simulink model "draft3"  (R2023a)
settings: Solver=VariableStepAuto  StartTime=0.0  StopTime=inf  FixedStep=0.0001  MaxStep=0.2  RelTol=1e-3  AbsTol=1e-3  EnableMultiTasking=on
model workspace (MAT data in the model file):
  c = 0.1
  k : Simulink.Parameter (value not decoded)
libraries: sm_lib x40, nesl_utility x35, simulink_extras x2, fl_lib x1
(part 3 of 3)

== system draft3/Thoracic Spine with rigid joints/T7 ==
  T7 : sm_lib/Body Elements/File Solid  ExtGeomFileName=C:\Users\siril\OneDrive\Desktop\TIM-Control\Matlab\Simscape models\CAD - with COM\T7_.step  UnitType=FromFile  ExtGeomFileUnits=m  StepReaderType=HEX  ExportConvexHullGeometry=off  InertiaType=CalculateFromGeometry  Mass=1  MassUnits=kg  CenterOfMass=[0 0 0]  CenterOfMassUnits=m  MomentsOfInertia=[1 1 1]  MomentsOfInertiaUnits=kg*m^2  ProductsOfInertia=[0 0 0]  ProductsOfInertiaUnits=kg*m^2  BasedOnType=Density  Density=0.99  DensityUnits=g/cm^3  DoExposeReferenceFrame=on  SerializedFrames=<Frames><Frame><Id>Frame1</Id><Value><Name>COM</Name><Origin><Source>CenterOfMassFrame</Source><FeatureName></FeatureName></Origin><PrimaryAxis><DefinedDirection>+Z</DefinedDirection><Source>ReferenceFrame</Source><SourceDirection>+Z</SourceDirection><FeatureName></FeatureName></PrimaryAxis><SecondaryAxis><DefinedDirection>+X</DefinedDirection><Source>ReferenceFrame</Source><SourceDirection>+X</SourceDirection><FeatureName></FeatureName></SecondaryAxis></Value></Frame><Frame><Id>Frame2</Id><Value><Name>to T8</Name><Origin><Source>GeometricFeature</Source><FeatureName>planar surface 5</FeatureName></Origin><PrimaryAxis><DefinedDirection>+X</DefinedDirection><Source>GeometricFeature</Source><SourceDirection>+Z</SourceDirection><FeatureName>planar surface 5</FeatureName></PrimaryAxis><SecondaryAxis><DefinedDirection>+Y</DefinedDirection><Source>ReferenceFrame</Source><SourceDirection>-X</SourceDirection><FeatureName></FeatureName></SecondaryAxis></Value></Frame><Frame><Id>Frame3</Id><Value><Name>to T6</Name><Origin><Source>GeometricFeature</Source><FeatureName>planar surface 10</FeatureName></Origin><PrimaryAxis><DefinedDirection>+Z</DefinedDirection><Source>ReferenceFrame</Source><SourceDirection>+Z</SourceDirection><FeatureName></FeatureName></PrimaryAxis><SecondaryAxis><DefinedDirection>+X</DefinedDirection><Source>ReferenceFrame</Source><SourceDirection>+X</SourceDirection><FeatureName></FeatureName></SecondaryAxis></Value></Frame></Frames>  GraphicType=FromGeometry  MarkerShape=Sphere  MarkerSize=10  GraphicVisPropType=SimpleVisualProperties  GraphicDiffuseColor=[0.5 0.5 0.5]  GraphicSpecularColor=[0.5 0.5 0.5 1.0]  GraphicAmbientColor=[0.15 0.15 0.15 1.0]  GraphicEmissiveColor=[0.0 0.0 0.0 1.0]  GraphicShininess=75  GraphicOpacity=1.0
  Weld Joint : sm_lib/Joints/Weld Joint  JointMode=Normal  SenseConstraintForce=off  SenseConstraintForceX=off  SenseConstraintForceY=off  SenseConstraintForceZ=off  SenseConstraintTorque=off  SenseConstraintTorqueX=off  SenseConstraintTorqueY=off  SenseConstraintTorqueZ=off  SenseTotalForce=off  SenseTotalForceX=off  SenseTotalForceY=off  SenseTotalForceZ=off  SenseTotalTorque=off  SenseTotalTorqueX=off  SenseTotalTorqueY=off  SenseTotalTorqueZ=off  CompositeWrenchDir=FollowerOnBase  CompositeWrenchFrame=BaseFrame
  to T8 : PMIOPort  Side=Left
  T7 COM : PMIOPort  Port=2  Side=Left
  T7 R : PMIOPort  Port=3  Side=Right
  to T6 : PMIOPort  Port=4  Side=Right
  connections:
  T7 COM/RConn1 -- T7/LConn1
  T7/RConn1 -- T7 R/RConn1
  to T6/RConn1 -- T7/RConn2
  to T8/RConn1 -- Weld Joint/LConn1
  Weld Joint/RConn1 -- T7/LConn2

== system draft3/Thoracic Spine with rigid joints/T8 ==
  T8 : sm_lib/Body Elements/File Solid  ExtGeomFileName=C:\Users\siril\OneDrive\Desktop\TIM-Control\Matlab\Simscape models\CAD - with COM\T8_.step  UnitType=FromFile  ExtGeomFileUnits=m  StepReaderType=HEX  ExportConvexHullGeometry=off  InertiaType=CalculateFromGeometry  Mass=1  MassUnits=kg  CenterOfMass=[0 0 0]  CenterOfMassUnits=m  MomentsOfInertia=[1 1 1]  MomentsOfInertiaUnits=kg*m^2  ProductsOfInertia=[0 0 0]  ProductsOfInertiaUnits=kg*m^2  BasedOnType=Density  Density=0.99  DensityUnits=g/cm^3  DoExposeReferenceFrame=on  SerializedFrames=<Frames><Frame><Id>Frame1</Id><Value><Name>COM</Name><Origin><Source>CenterOfMassFrame</Source><FeatureName></FeatureName></Origin><PrimaryAxis><DefinedDirection>+Z</DefinedDirection><Source>ReferenceFrame</Source><SourceDirection>+Z</SourceDirection><FeatureName></FeatureName></PrimaryAxis><SecondaryAxis><DefinedDirection>+X</DefinedDirection><Source>ReferenceFrame</Source><SourceDirection>+X</SourceDirection><FeatureName></FeatureName></SecondaryAxis></Value></Frame><Frame><Id>Frame2</Id><Value><Name>to T9</Name><Origin><Source>GeometricFeature</Source><FeatureName>planar surface 5</FeatureName></Origin><PrimaryAxis><DefinedDirection>+X</DefinedDirection><Source>GeometricFeature</Source><SourceDirection>+Z</SourceDirection><FeatureName>planar surface 5</FeatureName></PrimaryAxis><SecondaryAxis><DefinedDirection>+Y</DefinedDirection><Source>ReferenceFrame</Source><SourceDirection>-X</SourceDirection><FeatureName></FeatureName></SecondaryAxis></Value></Frame><Frame><Id>Frame3</Id><Value><Name>to T7</Name><Origin><Source>GeometricFeature</Source><FeatureName>planar surface 20</FeatureName></Origin><PrimaryAxis><DefinedDirection>+X</DefinedDirection><Source>GeometricFeature</Source><SourceDirection>+Z</SourceDirection><FeatureName>planar surface 20</FeatureName></PrimaryAxis><SecondaryAxis><DefinedDirection>+Y</DefinedDirection><Source>ReferenceFrame</Source><SourceDirection>-X</SourceDirection><FeatureName></FeatureName></SecondaryAxis></Value></Frame></Frames>  GraphicType=FromGeometry  MarkerShape=Sphere  MarkerSize=10  GraphicVisPropType=SimpleVisualProperties  GraphicDiffuseColor=[0.5 0.5 0.5]  GraphicSpecularColor=[0.5 0.5 0.5 1.0]  GraphicAmbientColor=[0.15 0.15 0.15 1.0]  GraphicEmissiveColor=[0.0 0.0 0.0 1.0]  GraphicShininess=75  GraphicOpacity=1.0
  Weld Joint : sm_lib/Joints/Weld Joint  JointMode=Normal  SenseConstraintForce=off  SenseConstraintForceX=off  SenseConstraintForceY=off  SenseConstraintForceZ=off  SenseConstraintTorque=off  SenseConstraintTorqueX=off  SenseConstraintTorqueY=off  SenseConstraintTorqueZ=off  SenseTotalForce=off  SenseTotalForceX=off  SenseTotalForceY=off  SenseTotalForceZ=off  SenseTotalTorque=off  SenseTotalTorqueX=off  SenseTotalTorqueY=off  SenseTotalTorqueZ=off  CompositeWrenchDir=FollowerOnBase  CompositeWrenchFrame=BaseFrame
  to T9 : PMIOPort  Side=Left
  T8 COM : PMIOPort  Port=2  Side=Left
  T8 R : PMIOPort  Port=3  Side=Right
  to T7 : PMIOPort  Port=4  Side=Right
  connections:
  to T7/RConn1 -- T8/RConn2
  T8/RConn1 -- T8 R/RConn1
  T8 COM/RConn1 -- T8/LConn1
  to T9/RConn1 -- Weld Joint/LConn1
  Weld Joint/RConn1 -- T8/LConn2

== system draft3/Thoracic Spine with rigid joints/T9 ==
  T9 : sm_lib/Body Elements/File Solid  ExtGeomFileName=C:\Users\siril\OneDrive\Desktop\TIM-Control\Matlab\Simscape models\CAD - with COM\T9_.step  UnitType=FromFile  ExtGeomFileUnits=m  StepReaderType=HEX  ExportConvexHullGeometry=off  InertiaType=CalculateFromGeometry  Mass=1  MassUnits=kg  CenterOfMass=[0 0 0]  CenterOfMassUnits=m  MomentsOfInertia=[1 1 1]  MomentsOfInertiaUnits=kg*m^2  ProductsOfInertia=[0 0 0]  ProductsOfInertiaUnits=kg*m^2  BasedOnType=Density  Density=0.99  DensityUnits=g/cm^3  DoExposeReferenceFrame=on  SerializedFrames=<Frames><Frame><Id>Frame1</Id><Value><Name>COM</Name><Origin><Source>CenterOfMassFrame</Source><FeatureName></FeatureName></Origin><PrimaryAxis><DefinedDirection>+Z</DefinedDirection><Source>ReferenceFrame</Source><SourceDirection>+Z</SourceDirection><FeatureName></FeatureName></PrimaryAxis><SecondaryAxis><DefinedDirection>+X</DefinedDirection><Source>ReferenceFrame</Source><SourceDirection>+X</SourceDirection><FeatureName></FeatureName></SecondaryAxis></Value></Frame><Frame><Id>Frame2</Id><Value><Name>to T10</Name><Origin><Source>GeometricFeature</Source><FeatureName>planar surface 5</FeatureName></Origin><PrimaryAxis><DefinedDirection>+X</DefinedDirection><Source>GeometricFeature</Source><SourceDirection>+Z</SourceDirection><FeatureName>planar surface 5</FeatureName></PrimaryAxis><SecondaryAxis><DefinedDirection>+Y</DefinedDirection><Source>ReferenceFrame</Source><SourceDirection>-X</SourceDirection><FeatureName></FeatureName></SecondaryAxis></Value></Frame><Frame><Id>Frame3</Id><Value><Name>to T8</Name><Origin><Source>GeometricFeature</Source><FeatureName>planar surface 15</FeatureName></Origin><PrimaryAxis><DefinedDirection>+X</DefinedDirection><Source>GeometricFeature</Source><SourceDirection>+Z</SourceDirection><FeatureName>planar surface 15</FeatureName></PrimaryAxis><SecondaryAxis><DefinedDirection>+Y</DefinedDirection><Source>ReferenceFrame</Source><SourceDirection>-X</SourceDirection><FeatureName></FeatureName></SecondaryAxis></Value></Frame></Frames>  GraphicType=FromGeometry  MarkerShape=Sphere  MarkerSize=10  GraphicVisPropType=SimpleVisualProperties  GraphicDiffuseColor=[0.5 0.5 0.5]  GraphicSpecularColor=[0.5 0.5 0.5 1.0]  GraphicAmbientColor=[0.15 0.15 0.15 1.0]  GraphicEmissiveColor=[0.0 0.0 0.0 1.0]  GraphicShininess=75  GraphicOpacity=1.0
  Weld Joint : sm_lib/Joints/Weld Joint  JointMode=Normal  SenseConstraintForce=off  SenseConstraintForceX=off  SenseConstraintForceY=off  SenseConstraintForceZ=off  SenseConstraintTorque=off  SenseConstraintTorqueX=off  SenseConstraintTorqueY=off  SenseConstraintTorqueZ=off  SenseTotalForce=off  SenseTotalForceX=off  SenseTotalForceY=off  SenseTotalForceZ=off  SenseTotalTorque=off  SenseTotalTorqueX=off  SenseTotalTorqueY=off  SenseTotalTorqueZ=off  CompositeWrenchDir=FollowerOnBase  CompositeWrenchFrame=BaseFrame
  to T10 : PMIOPort  Side=Left
  T9 COM : PMIOPort  Port=2  Side=Left
  T9 R : PMIOPort  Port=3  Side=Right
  to T8 : PMIOPort  Port=4  Side=Right
  connections:
  T9 COM/RConn1 -- T9/LConn1
  T9/RConn1 -- T9 R/RConn1
  to T8/RConn1 -- T9/RConn2
  to T10/RConn1 -- Weld Joint/LConn1
  Weld Joint/RConn1 -- T9/LConn2

== matlab function draft3/L1/LB torque feedback L4/peacewise torque profile4 ==
  data: u input; torque output
function torque = T(u)
torque = 0;
if (u >= 15)
    torque= -0.0015*1*(57.295*15)^4 + 0.1326*(57.295*15)^3 -0.3477*(57.295*15)^2 + 0.499*(57.295*15);
 
elseif (u >= -15 && u<= 15)
    torque= -0.0015*(57.295*u)^4 + 0.1326*(57.295*u)^3 -0.3477*(57.295*u)^2 + 0.499*(57.295*u)   ;
    
elseif (u <= -15)
   torque= -0.0015*1*(57.295*-15)^4 + 0.1326*(57.295*-15)^3 -0.3477*(57.295*-15)^2 + 0.499*(57.295*-15);
end

== matlab function draft3/L5/FE torque feedback L5/peacewise torque profile (+- 15 deg) ==
  data: u input; torque output
function torque = T(u)
torque = 0;
if (u >= 15)
    torque= -0.0015*1*(57.295*15)^4 + 0.1326*(57.295*15)^3 -0.3477*(57.295*15)^2 + 0.499*(57.295*15);
 
elseif (u >= -15 && u<= 15)
    torque= -0.0015*(57.295*u)^4 + 0.1326*(57.295*u)^3 -0.3477*(57.295*u)^2 + 0.499*(57.295*u)   ;
    
elseif (u <= -15)
   torque= -0.0015*1*(57.295*-15)^4 + 0.1326*(57.295*-15)^3 -0.3477*(57.295*-15)^2 + 0.499*(57.295*-15);
end

== matlab function draft3/L5/LB torque feedback L5/peacewise torque profile2 ==
  data: u input; torque output
function torque = T(u)
torque = 0;
if (u >= 15)
    torque= -0.0015*1*(57.295*15)^4 + 0.1326*(57.295*15)^3 -0.3477*(57.295*15)^2 + 0.499*(57.295*15);
 
elseif (u >= -15 && u<= 15)
    torque= -0.0015*(57.295*u)^4 + 0.1326*(57.295*u)^3 -0.3477*(57.295*u)^2 + 0.499*(57.295*u)   ;
    
elseif (u <= -15)
   torque= -0.0015*1*(57.295*-15)^4 + 0.1326*(57.295*-15)^3 -0.3477*(57.295*-15)^2 + 0.499*(57.295*-15);
end

== matlab function draft3/L5/AR torque feedback L5/peacewise torque profile3 ==
  data: u input; torque output
function torque = T(u)
torque = 0;
if (u >= 15)
    torque= -0.0015*1*(57.295*15)^4 + 0.1326*(57.295*15)^3 -0.3477*(57.295*15)^2 + 0.499*(57.295*15);
 
elseif (u >= -15 && u<= 15)
    torque= -0.0015*(57.295*u)^4 + 0.1326*(57.295*u)^3 -0.3477*(57.295*u)^2 + 0.499*(57.295*u)   ;
    
elseif (u <= -15)
   torque= -0.0015*1*(57.295*-15)^4 + 0.1326*(57.295*-15)^3 -0.3477*(57.295*-15)^2 + 0.499*(57.295*-15);
end

== matlab function draft3/L4/LB torque feedback L4/peacewise torque profile4 ==
  data: u input; torque output
function torque = T(u)
torque = 0;
if (u >= 15)
    torque= -0.0015*1*(57.295*15)^4 + 0.1326*(57.295*15)^3 -0.3477*(57.295*15)^2 + 0.499*(57.295*15);
 
elseif (u >= -15 && u<= 15)
    torque= -0.0015*(57.295*u)^4 + 0.1326*(57.295*u)^3 -0.3477*(57.295*u)^2 + 0.499*(57.295*u)   ;
    
elseif (u <= -15)
   torque= -0.0015*1*(57.295*-15)^4 + 0.1326*(57.295*-15)^3 -0.3477*(57.295*-15)^2 + 0.499*(57.295*-15);
end

== matlab function draft3/L4/AR torque feedback L4/peacewise torque profile5 ==
  data: u input; torque output
function torque = T(u)
torque = 0;
if (u >= 15)
    torque= -0.0015*1*(57.295*15)^4 + 0.1326*(57.295*15)^3 -0.3477*(57.295*15)^2 + 0.499*(57.295*15);
 
elseif (u >= -15 && u<= 15)
    torque= -0.0015*(57.295*u)^4 + 0.1326*(57.295*u)^3 -0.3477*(57.295*u)^2 + 0.499*(57.295*u)   ;
    
elseif (u <= -15)
   torque= -0.0015*1*(57.295*-15)^4 + 0.1326*(57.295*-15)^3 -0.3477*(57.295*-15)^2 + 0.499*(57.295*-15);
end

== matlab function draft3/L3/AR torque feedback L4/peacewise torque profile5 ==
  data: u input; torque output
function torque = T(u)
torque = 0;
if (u >= 15)
    torque= -0.0015*1*(57.295*15)^4 + 0.1326*(57.295*15)^3 -0.3477*(57.295*15)^2 + 0.499*(57.295*15);
 
elseif (u >= -15 && u<= 15)
    torque= -0.0015*(57.295*u)^4 + 0.1326*(57.295*u)^3 -0.3477*(57.295*u)^2 + 0.499*(57.295*u)   ;
    
elseif (u <= -15)
   torque= -0.0015*1*(57.295*-15)^4 + 0.1326*(57.295*-15)^3 -0.3477*(57.295*-15)^2 + 0.499*(57.295*-15);
end

== matlab function draft3/L3/FE torque feedback L4/peacewise torque profile1 ==
  data: u input; torque output
function torque = T(u)
torque = 0;
if (u >= 15)
    torque= -0.0015*1*(57.295*15)^4 + 0.1326*(57.295*15)^3 -0.3477*(57.295*15)^2 + 0.499*(57.295*15);
 
elseif (u >= -15 && u<= 15)
    torque= -0.0015*(57.295*u)^4 + 0.1326*(57.295*u)^3 -0.3477*(57.295*u)^2 + 0.499*(57.295*u)   ;
    
elseif (u <= -15)
   torque= -0.0015*1*(57.295*-15)^4 + 0.1326*(57.295*-15)^3 -0.3477*(57.295*-15)^2 + 0.499*(57.295*-15);
end

== matlab function draft3/L3/LB torque feedback L4/peacewise torque profile4 ==
  data: u input; torque output
function torque = T(u)
torque = 0;
if (u >= 15)
    torque= -0.0015*1*(57.295*15)^4 + 0.1326*(57.295*15)^3 -0.3477*(57.295*15)^2 + 0.499*(57.295*15);
 
elseif (u >= -15 && u<= 15)
    torque= -0.0015*(57.295*u)^4 + 0.1326*(57.295*u)^3 -0.3477*(57.295*u)^2 + 0.499*(57.295*u)   ;
    
elseif (u <= -15)
   torque= -0.0015*1*(57.295*-15)^4 + 0.1326*(57.295*-15)^3 -0.3477*(57.295*-15)^2 + 0.499*(57.295*-15);
end

== matlab function draft3/L4/FE torque feedback L4/peacewise torque profile1 ==
  data: u input; torque output
function torque = T(u)
torque = 0;
if (u >= 15)
    torque= -0.0015*1*(57.295*15)^4 + 0.1326*(57.295*15)^3 -0.3477*(57.295*15)^2 + 0.499*(57.295*15);
 
elseif (u >= -15 && u<= 15)
    torque= -0.0015*(57.295*u)^4 + 0.1326*(57.295*u)^3 -0.3477*(57.295*u)^2 + 0.499*(57.295*u)   ;
    
elseif (u <= -15)
   torque= -0.0015*1*(57.295*-15)^4 + 0.1326*(57.295*-15)^3 -0.3477*(57.295*-15)^2 + 0.499*(57.295*-15);
end

== matlab function draft3/L2/AR torque feedback L4/peacewise torque profile5 ==
  data: u input; torque output
function torque = T(u)
torque = 0;
if (u >= 15)
    torque= -0.0015*1*(57.295*15)^4 + 0.1326*(57.295*15)^3 -0.3477*(57.295*15)^2 + 0.499*(57.295*15);
 
elseif (u >= -15 && u<= 15)
    torque= -0.0015*(57.295*u)^4 + 0.1326*(57.295*u)^3 -0.3477*(57.295*u)^2 + 0.499*(57.295*u)   ;
    
elseif (u <= -15)
   torque= -0.0015*1*(57.295*-15)^4 + 0.1326*(57.295*-15)^3 -0.3477*(57.295*-15)^2 + 0.499*(57.295*-15);
end

== matlab function draft3/L2/FE torque feedback L4/peacewise torque profile1 ==
  data: u input; torque output
function torque = T(u)
torque = 0;
if (u >= 15)
    torque= -0.0015*1*(57.295*15)^4 + 0.1326*(57.295*15)^3 -0.3477*(57.295*15)^2 + 0.499*(57.295*15);
 
elseif (u >= -15 && u<= 15)
    torque= -0.0015*(57.295*u)^4 + 0.1326*(57.295*u)^3 -0.3477*(57.295*u)^2 + 0.499*(57.295*u)   ;
    
elseif (u <= -15)
   torque= -0.0015*1*(57.295*-15)^4 + 0.1326*(57.295*-15)^3 -0.3477*(57.295*-15)^2 + 0.499*(57.295*-15);
end

== matlab function draft3/L2/LB torque feedback L4/peacewise torque profile4 ==
  data: u input; torque output
function torque = T(u)
torque = 0;
if (u >= 15)
    torque= -0.0015*1*(57.295*15)^4 + 0.1326*(57.295*15)^3 -0.3477*(57.295*15)^2 + 0.499*(57.295*15);
 
elseif (u >= -15 && u<= 15)
    torque= -0.0015*(57.295*u)^4 + 0.1326*(57.295*u)^3 -0.3477*(57.295*u)^2 + 0.499*(57.295*u)   ;
    
elseif (u <= -15)
   torque= -0.0015*1*(57.295*-15)^4 + 0.1326*(57.295*-15)^3 -0.3477*(57.295*-15)^2 + 0.499*(57.295*-15);
end

== matlab function draft3/L1/AR torque feedback L4/peacewise torque profile5 ==
  data: u input; torque output
function torque = T(u)
torque = 0;
if (u >= 15)
    torque= -0.0015*1*(57.295*15)^4 + 0.1326*(57.295*15)^3 -0.3477*(57.295*15)^2 + 0.499*(57.295*15);
 
elseif (u >= -15 && u<= 15)
    torque= -0.0015*(57.295*u)^4 + 0.1326*(57.295*u)^3 -0.3477*(57.295*u)^2 + 0.499*(57.295*u)   ;
    
elseif (u <= -15)
   torque= -0.0015*1*(57.295*-15)^4 + 0.1326*(57.295*-15)^3 -0.3477*(57.295*-15)^2 + 0.499*(57.295*-15);
end

== matlab function draft3/L1/FE torque feedback L4/peacewise torque profile1 ==
  data: u input; torque output
function torque = T(u)
torque = 0;
if (u >= 15)
    torque= -0.0015*1*(57.295*15)^4 + 0.1326*(57.295*15)^3 -0.3477*(57.295*15)^2 + 0.499*(57.295*15);
 
elseif (u >= -15 && u<= 15)
    torque= -0.0015*(57.295*u)^4 + 0.1326*(57.295*u)^3 -0.3477*(57.295*u)^2 + 0.499*(57.295*u)   ;
    
elseif (u <= -15)
   torque= -0.0015*1*(57.295*-15)^4 + 0.1326*(57.295*-15)^3 -0.3477*(57.295*-15)^2 + 0.499*(57.295*-15);
end
